simulink model "bai29"  (R2014a)
settings: Solver=ode45  StartTime=1.0  StopTime=10.0  RelTol=1e-3
settings Model: Creator=Lan  LastModifiedBy=Lan

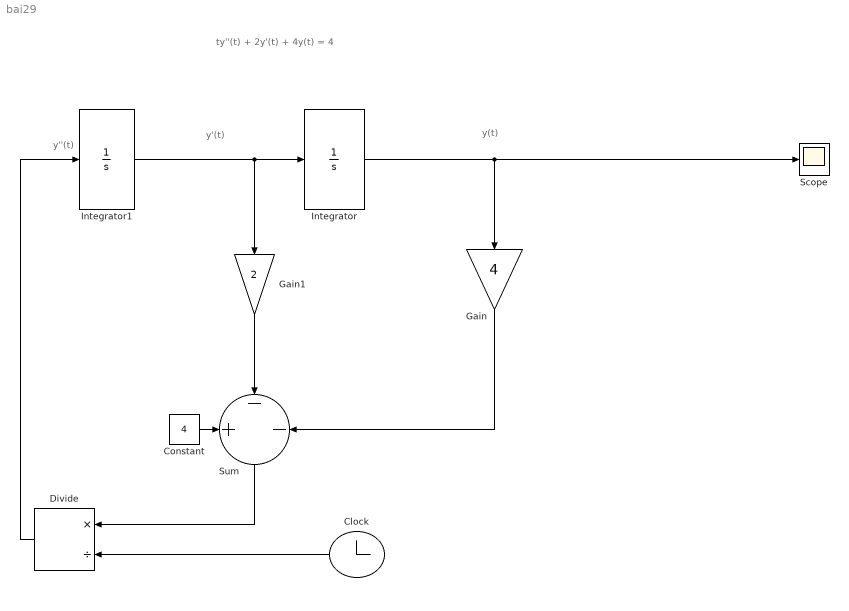
== system bai29 ==
  note: y(t)
  note: y'(t)
  note: y''(t)
  note: ty''(t) + 2y'(t) + 4y(t) = 4
  Clock : Clock
  Constant : Constant  Value=4
  Divide : Product  Inputs=*/
  Gain : Gain  Gain=4
  Gain1 : Gain  Gain=2
  Integrator : Integrator  InitialCondition=1
  Integrator1 : Integrator  InitialCondition=1
  Scope : Scope
  Sum : Sum  Inputs=+--
  wires:
  Integrator1/1 -> Integrator/1, Gain1/1
  Integrator/1 -> Scope/1, Gain/1
  Gain1/1 -> Sum/2
  Gain/1 -> Sum/3
  Constant/1 -> Sum/1
  Sum/1 -> Divide/1
  Clock/1 -> Divide/2
  Divide/1 -> Integrator1/1
